simulink model "Task_15"  (R2022b)
settings: Solver=VariableStepAuto  StartTime=0.0  StopTime=10.0  RelTol=1e-3
settings Model: Creator=Abanob_Sameh  LastModifiedBy=Abanob_Sameh

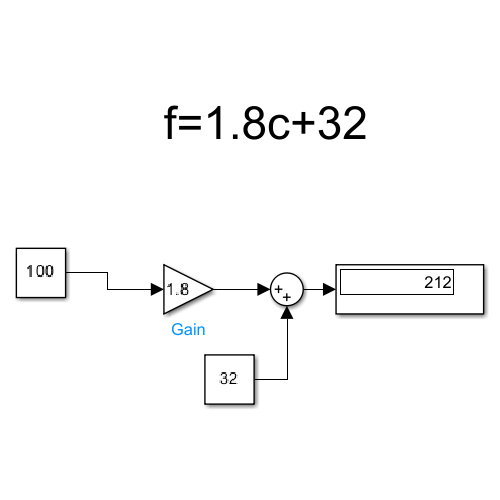
[thumbnail: Simulink's stored preview of the top-level diagram]
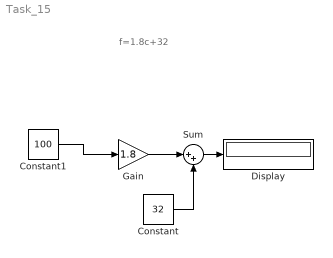
== system Task_15 ==
  note: f=1.8c+32
  Constant : Constant  Value=32
  Constant1 : Constant  Value=100
  Display : Display
  Gain : Gain  Gain=1.8
  Sum : Sum  Inputs=|++
  wires:
  Constant1/1 -> Gain/1
  Gain/1 -> Sum/1
  Constant/1 -> Sum/2
  Sum/1 -> Display/1
